simulink model "q_as_mpc"  (R2019a)
settings: Solver=ode1  StartTime=0.0  StopTime=inf  FixedStep=0.001  RelTol=1e-3  EnableMultiTasking=on
values from neighbouring files (symbols this model uses):
  A = [ 0 1 0 -1 ... (first row only)    [setup_as.m]
  B = [0  0 ; 0 1/ms ; -1  0 ; bus/mu -1/mu ]    [setup_as.m]
  C = [ 1 0 0 0 ; -ks/ms -bs/ms 0 bs/ms]    [setup_as.m]
  D = zeros(2,2); D(2,2)=1/ms    [setup_as.m]
  K = lqr( A, B(:,2), Q, R )    [setup_as.m]
  umax = -umin    (= 30)    [setup_as.m]
  umin = -30    [setup_as.m]
  wt_u = R    [setup_as.m]
  wt_y = diag(Q)'    [setup_as.m]
  ymax = -ymin    [setup_as.m]
undefined symbols (not defined in the file or in its folder): HIL, K_d, K_p, qc_get_step_size, ymin
libraries: quarc_library x9, simulink x3, mpclib x2
settings Model: SimulationMode=external  ExtModeTrigDuration=50000  Creator=DCrymble  LastModifiedBy=jxs210080
settings SolverCC: PositivePriorityOrder=on  AutoInsertRateTranBlk=on
settings DataIOCC: LimitDataPoints=on  SaveFormat=Array  SignalLoggingSaveFormat=ModelDataLogs  ReturnWorkspaceOutputs=off
settings OptimizationCC: BooleanDataType=off  OptimizeBlockIOStorage=off  BufferReuse=off  GlobalBufferReuse=off  ExpressionFolding=off  ExpressionDepthLimit=2147483647  LocalBlockOutputs=off  InitFltsAndDblsToZero=on  LifeSpan=inf  OptimizeDataStoreBuffers=off  BusAssignmentInplaceUpdate=off
settings DebuggingCC: UnderspecifiedInitializationDetection=Classic  MergeDetectMultiDrivingBlocksExec=none  SolverPrmCheckMsg=warning  FcnCallInpInsideContextMsg=warning  StateNameClashWarn=warning  SFUnexpectedBacktrackingDiag=warning  SFNoUnconditionalDefaultTransitionDiag=warning  ArithmeticOperatorsInVariantConditions=warning
settings HardwareCC: ProdBitPerPointer=32  ProdBitPerSizeT=32  ProdBitPerPtrDiffT=32  ProdLargestAtomicFloat=None  ProdIntDivRoundTo=Undefined  ProdEndianess=Unspecified  ProdWordSize=32  ProdHWDeviceType=32-bit Generic
settings ModelReferenceCC: PropagateSignalLabelsOutOfModel=off
settings SFSimCC: SimUseLocalCustomCode=off  SimParseCustomCode=off
settings RTWCC: SystemTargetFile=quarc_windows.tlc  TemplateMakefile=quarc_default_tmf  Description=QuaRC Win32 Target  RTWUseLocalCustomCode=off
settings CodeAppCC: StateflowObjectComments=on
settings STFCustomTargetCC: TargetPreCompLibLocation=C:\PROGRA~3\QUARC\lib\2019a\windows\release  ConcurrentExecutionCompliant=on  GeneratePreprocessorConditionals=Disable all  CPPClassGenCompliant=on  SystemTargetFile=quarc_windows.tlc
settings GRTTargetCC: TargetPreCompLibLocation=C:\PROGRA~3\QUARC\lib\2019a\windows\release  TargetLangStandard=C89/C90 (ANSI)  ParMdlRefBuildCompliant=off  CompOptLevelCompliant=off  GeneratePreprocessorConditionals=Disable all  CombineOutputUpdateFcns=off  MatFileLogging=off  GRTInterface=on  UseToolchainInfoCompliant=off  ExtMode=on  ExtModeMexFile=quarc_comm
settings ConfigComp: CovMetricSettings=dw  CovHtmlReporting=on  CovSaveCumulativeToWorkspaceVar=on  CovSaveSingleToWorkspaceVar=on  CovExternalEMLEnable=off

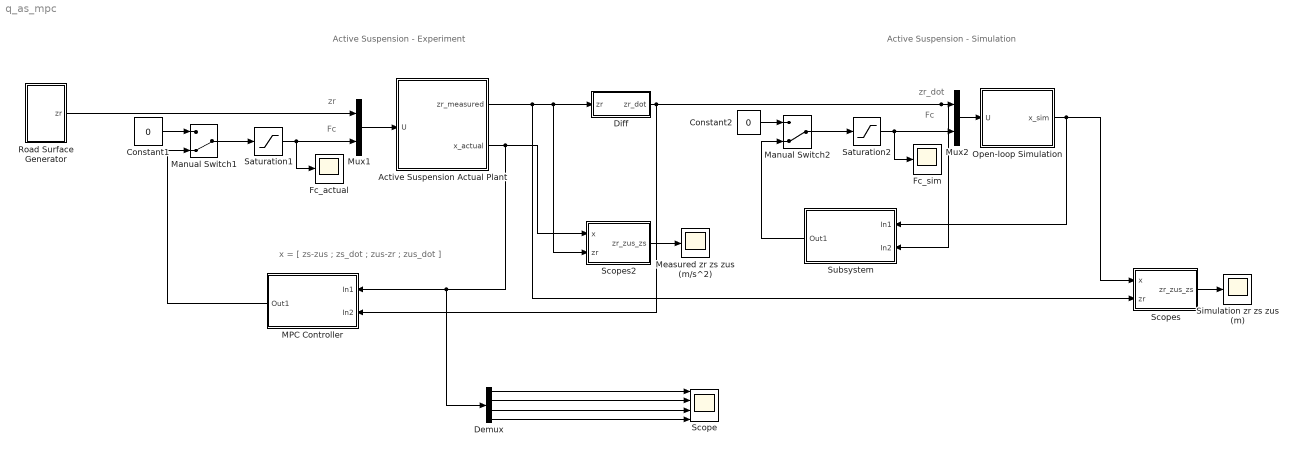
== system q_as_mpc ==
  note: Active Suspension - Experiment
  note: zr
  note: Fc
  note: zr_dot
  note: Fc
  note: x = [ zs-zus ; zs_dot ; zus-zr ; zus_dot ]
  note: Active Suspension - Simulation
  Active Suspension Actual Plant : Subsystem
  Constant1 : Constant  Value=0
  Constant2 : Constant  Value=0
  Demux : Demux
  Diff : Subsystem
  Fc_actual : Scope
  Fc_sim : Scope
  MPC Controller : Subsystem  VariantControl=Variant1
  Manual Switch1 : ManualSwitch  CurrentSetting=0
  Manual Switch2 : ManualSwitch  CurrentSetting=0
  Measured zr zs zus (m/s^2) : Scope
  Mux1 : Mux  Inputs=2
  Mux2 : Mux  Inputs=2
  Open-loop Simulation : Subsystem
  Road Surface Generator : Subsystem
  Saturation1 : Saturate  UpperLimit=38.3  LowerLimit=-38.3
  Saturation2 : Saturate  UpperLimit=39.2  LowerLimit=-39.2
  Scope : Scope  NumInputPorts=4
  Scopes : Subsystem
  Scopes2 : Subsystem
  Simulation zr zs zus (m) : Scope
  Subsystem : Subsystem  VariantControl=Variant1
  wires:
  Road Surface Generator/1(zr) -> Mux1/1
  Manual Switch1/1 -> Saturation1/1
  Mux1/1 -> Active Suspension Actual Plant/1(U)
  Constant1/1 -> Manual Switch1/1
  Saturation1/1 -> Fc_actual/1, Mux1/2
  Constant2/1 -> Manual Switch2/1
  Manual Switch2/1 -> Saturation2/1
  Mux2/1 -> Open-loop Simulation/1(U)
  Scopes2/1(zr_zus_zs) -> Measured zr zs zus (m/s^2)/1
  Scopes/1(zr_zus_zs) -> Simulation zr zs zus (m)/1
  Saturation2/1 -> Mux2/2, Fc_sim/1
  MPC Controller/1(Out1) -> Manual Switch1/2
  Active Suspension Actual Plant/1(zr_measured) -> Scopes/2(zr), Diff/1(zr), Scopes2/2(zr)
  Open-loop Simulation/1(x_sim) -> Subsystem/1(In1), Scopes/1(x)
  Diff/1(zr_dot) -> Subsystem/2(In2), Mux2/1, MPC Controller/2(In2)
  Subsystem/1(Out1) -> Manual Switch2/2
  Active Suspension Actual Plant/2(x_actual) -> Demux/1, MPC Controller/1(In1), Scopes2/1(x)
  Demux/1 -> Scope/1
  Demux/2 -> Scope/2
  Demux/3 -> Scope/3
  Demux/4 -> Scope/4

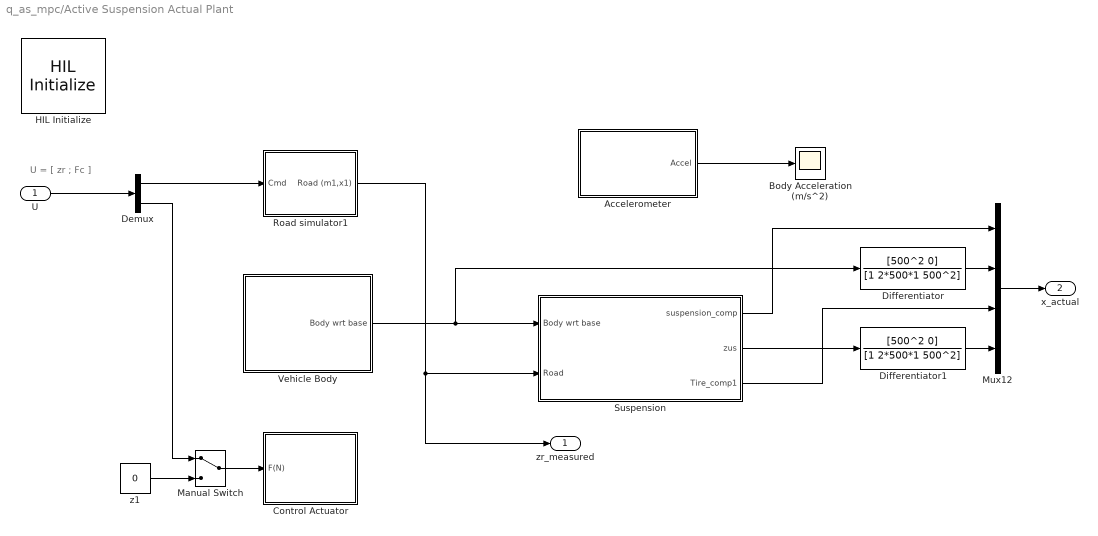
== system q_as_mpc/Active Suspension Actual Plant ==
  note: U = [ zr ; Fc ]
  U : Inport
  Accelerometer : Subsystem
  Body Acceleration (m/s^2) : Scope
  Control Actuator : Subsystem
  Demux : Demux  Outputs=2
  Differentiator : TransferFcn  Numerator=[500^2 0]  Denominator=[1 2*500*1 500^2]
  Differentiator1 : TransferFcn  Numerator=[500^2 0]  Denominator=[1 2*500*1 500^2]
  HIL Initialize : quarc_library/Data Acquisition/Generic/Configuration/HIL Initialize  Priority=-99  object_name=HIL-1  board_type=q8_usb  board_number=0  board_options=update_rate=normal;decimation=1  exclusive=off  active=off  hardware_clocks=[0:2]  clock_modes=[]  initial_clock_frequencies=[]  set_clock_params_at_start=off  set_clock_params_at_switch_in=off  set_clock_frequencies_at_start=off  set_clock_frequencies_at_switch_in=off  analog_input_channels=[0:7]  analog_input_configurations=[]  analog_input_maximums=10  analog_input_minimums=-10  set_analog_input_params_at_start=on  set_analog_input_params_at_switch_in=off  analog_output_channels=[0:7]  analog_output_maximums=10  analog_output_minimums=-10  initial_analog_outputs=[0]  final_analog_outputs=[0]  watchdog_analog_outputs=0  set_analog_output_params_at_start=on  set_analog_output_params_at_switch_in=off  set_analog_outputs_at_start=on  set_analog_outputs_at_switch_in=off  set_analog_outputs_at_terminate=on  set_analog_outputs_at_switch_out=off  set_analog_outputs_on_watchdog=off  digital_input_channels=[]  digital_output_channels=[0:4]  digital_output_configuration=[]  initial_digital_outputs=[0 0 0 0 1]  final_digital_outputs=[1 1 1 1 0]  watchdog_digital_outputs=1  set_digital_output_params_at_start=off  set_digital_output_params_at_switch_in=off  set_digital_outputs_at_start=on  set_digital_outputs_at_switch_in=off  set_digital_outputs_at_terminate=on  set_digital_outputs_at_switch_out=off  set_digital_outputs_on_watchdog=off  encoder_channels=[0:7]  quadrature=[4]  encoder_filter_frequency=[]  initial_encoder_counts=[0]  set_encoder_params_at_start=on  set_encoder_params_at_switch_in=off  set_encoder_counts_at_start=on  set_encoder_counts_at_switch_in=off  pwm_channels=[0:7]  pwm_modes=0  pwm_frequency=99.532799999999995e6/4095  pwm_configuration=[0]  pwm_alignment=[0]  pwm_polarity=[1]  pwm_leading_deadband=[0]  pwm_trailing_deadband=[0]  initial_pwm_outputs=[0]  final_pwm_outputs=[0]  watchdog_pwm_outputs=[0]  set_pwm_params_at_start=on  set_pwm_params_at_switch_in=off  set_pwm_outputs_at_start=on  set_pwm_outputs_at_switch_in=off  set_pwm_outputs_at_terminate=on  set_pwm_outputs_at_switch_out=off  set_pwm_outputs_on_watchdog=off  other_output_channels=[]  initial_other_outputs=[]  final_other_outputs=[]  watchdog_other_outputs=[]  set_other_outputs_at_start=off  set_other_outputs_at_switch_in=off  set_other_outputs_at_terminate=off  set_other_outputs_at_switch_out=off  set_other_outputs_on_watchdog=off
  Manual Switch : ManualSwitch
  Mux12 : Mux
  Road simulator1 : Subsystem
  Suspension : Subsystem
  Vehicle Body : Subsystem
  z1 : Constant  Value=0
  zr_measured : Outport
  x_actual : Outport  Port=2
  wires:
  Manual Switch/1 -> Control Actuator/1(F(N))
  z1/1 -> Manual Switch/2
  Suspension/1(suspension_comp) -> Mux12/1
  Vehicle Body/1(Body wrt base) -> Differentiator/1, Suspension/1("Body wrt base ")
  Differentiator/1 -> Mux12/2
  Differentiator1/1 -> Mux12/4
  Suspension/2(zus) -> Differentiator1/1
  Mux12/1 -> x_actual/1
  Suspension/3(Tire_comp1) -> Mux12/3
  U/1 -> Demux/1
  Road simulator1/1(Road (m1,x1)) -> zr_measured/1, Suspension/2(Road)
  Demux/1 -> Road simulator1/1(Cmd)
  Demux/2 -> Manual Switch/1
  Accelerometer/1(Accel) -> Body Acceleration (m/s^2)/1

== system q_as_mpc/Diff ==
  zr : Inport
  2nd Order Filter Input ICs3 : Subsystem
  Constant3 : Constant  Value=1000
  Terminator_1 : Terminator
  z4 : Constant
  zr_dot : Outport
  wires:
  Constant3/1 -> 2nd Order Filter Input ICs3/2(Wn)
  z4/1 -> 2nd Order Filter Input ICs3/3(z)
  zr/1 -> 2nd Order Filter Input ICs3/1(In)
  2nd Order Filter Input ICs3/2(Out_dot) -> zr_dot/1
  2nd Order Filter Input ICs3/1(Out) -> Terminator_1/1

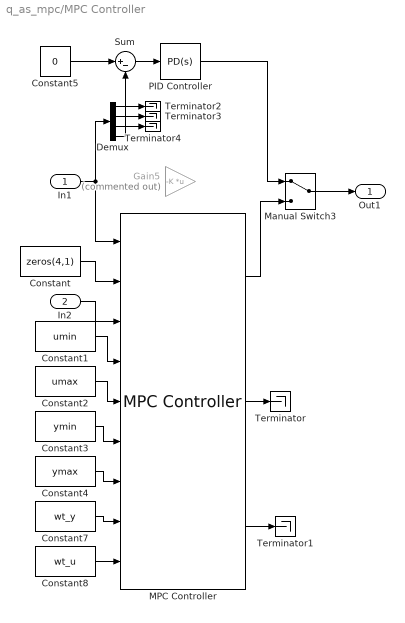
== system q_as_mpc/MPC Controller ==
  In1 : Inport
  In2 : Inport  Port=2
  Constant : Constant  Value=zeros(4,1)
  Constant1 : Constant  Value=umin
  Constant2 : Constant  Value=umax
  Constant3 : Constant  Value=ymin
  Constant4 : Constant  Value=ymax
  Constant5 : Constant  Value=0
  Constant7 : Constant  Value=wt_y
  Constant8 : Constant  Value=wt_u
  Demux : Demux
  Gain5 : Gain  Commented=on  Gain=-K  Multiplication=Matrix(K*u)
  MPC Controller : mpclib/MPC Controller  SCDEnableBlockLinearizationSpecification=on  mpcobj=ctr_mpc  is_multiple=0  enable_value=0  return_u0=off  updateMPCinCallerWorkspace=on  md_inport=on  mv_inport=off  uref_inport=off  return_cost=off  return_mvseq=on  return_qpstatus=off  return_xseq=off  return_state=off  return_ovseq=on  state_inport=off  umin_inport=on  umax_inport=on  ymin_inport=on  ymax_inport=on  cc_inport=off  ywt_inport=on  uwt_inport=on  duwt_inport=off  rhoeps_inport=off  pm_inport=off  MaximumP=100  HorizonChoice=FixedHorizon  n_ts=0.01  n_p=20  n_mv=1  n_md=1  n_ud=0  n_mo=4  n_uo=0  BlockDataType=double  SampleTimeInherited=off  switch_inport=off
      settings: SourceProductName=MATLAB Runtime - Model Predictive Control Toolbox Addin  SourceProductBaseCode=Missing
  Manual Switch3 : ManualSwitch
  PID Controller : simulink/Continuous/PID Controller  Controller=PD  Form=Parallel  TimeDomain=Continuous-time  SampleTime=-1  IntegratorMethod=Forward Euler  FilterMethod=Forward Euler  ControllerParametersSource=internal  P=K_p  I=1  D=K_d  UseFilter=on  N=100  TunerSelectOption=Transfer Function Based (PID Tuner App)  InitialConditionSource=internal  InitialConditionForIntegrator=0  InitialConditionForFilter=0  DifferentiatorICPrevScaledInput=0  ExternalReset=none  TrackingMode=off  Kt=1  LimitOutput=off  UpperSaturationLimit=inf  LowerSaturationLimit=-inf  LinearizeAsGain=on  AntiWindupMode=none  Kb=1  POutMin=[]  POutMax=[]  IOutMin=[]  IOutMax=[]  DOutMin=[]  DOutMax=[]  NOutMin=[]  NOutMax=[]  SumOutMin=[]  SumOutMax=[]  SaturationOutMin=[]  SaturationOutMax=[]  PParamMin=[]  PParamMax=[]  IParamMin=[]  IParamMax=[]  DParamMin=[]  DParamMax=[]  NParamMin=[]  NParamMax=[]  KbParamMin=[]  KbParamMax=[]  KtParamMin=[]  KtParamMax=[]  KbOutMin=[]  KbOutMax=[]  KtOutMin=[]  KtOutMax=[]  IntegratorOutMin=[]  IntegratorOutMax=[]  FilterOutMin=[]  FilterOutMax=[]  SumI1OutMin=[]  SumI1OutMax=[]  SumI2OutMin=[]  SumI2OutMax=[]  SumI3OutMin=[]  SumI3OutMax=[]  SumI4OutMin=[]  SumI4OutMax=[]  SumDOutMin=[]  SumDOutMax=[]  DifferentiatorOutMin=[]  DifferentiatorOutMax=[]  FilterDiffOutCoefMin=[]  FilterDiffOutCoefMax=[]  ReciprocalOutMin=[]  ReciprocalOutMax=[]  SumDenOutMin=[]  SumDenOutMax=[]  SumNumOutMin=[]  SumNumOutMax=[]  DivideOutMin=[]  DivideOutMax=[]  IntegratorContinuousStateAttributes=''  IntegratorStateMustResolveToSignalObject=off  IntegratorRTWStateStorageClass=Auto  FilterContinuousStateAttributes=''  FilterStateMustResolveToSignalObject=off  FilterRTWStateStorageClass=Auto  ParallelPVariant=InternalParameters  IdealPVariant=Disabled  IVariant=Disabled  DVariant=InternalParameters  IntegratorVariant=Disabled  SatVariant=Disabled  AWVariant=Disabled  PCopyVariant=Disabled  TRVariant=Disabled  FdbkBlocksVariant=Forward  IdealPFdbkVariant=Disabled  SatFdbkVariant=Disabled  DerivativeFilterVariant=ContFilter  NVariant=InternalParameters  NCopyVariant=Disabled  FilterICVariant=InternalICsFilter  IntegratorICVariant=Disabled  ExternalResetVariant=Disabled  TRSumVariant=Passthrough  SumFdbkVariant=Disabled  SumVariant=Sum_PD
  Sum : Sum  Inputs=|+-
  Terminator{,1..4} (5 alike) : Terminator
  Out1 : Outport
  wires:
  In2/1 -> MPC Controller/3
  Constant1/1 -> MPC Controller/4
  Manual Switch3/1 -> Out1/1
  Constant8/1 -> MPC Controller/9
  Constant7/1 -> MPC Controller/8
  Constant4/1 -> MPC Controller/7
  Constant3/1 -> MPC Controller/6
  Constant2/1 -> MPC Controller/5
  In1/1 -> Demux/1, MPC Controller/1
  Constant/1 -> MPC Controller/2
  MPC Controller/1 -> Manual Switch3/2
  MPC Controller/2 -> Terminator/1
  MPC Controller/3 -> Terminator1/1
  Constant5/1 -> Sum/1
  Sum/1 -> PID Controller/1
  Demux/4 -> Sum/2
  PID Controller/1 -> Manual Switch3/1
  Demux/1 -> Terminator2/1
  Demux/2 -> Terminator3/1
  Demux/3 -> Terminator4/1

== system q_as_mpc/Open-loop Simulation ==
  U : Inport
  Demux : Demux  Outputs=[4 2]
  Open-Loop State-Space : StateSpace  A=A  B=B  C=cat(1,eye(4), C)  D=cat(1,zeros(4,2),D)  InitialCondition=0
  Terminator : Terminator
  Unit Delay : UnitDelay  SampleTime=-1  HasFrameUpgradeWarning=on
  x_sim : Outport
  wires:
  Open-Loop State-Space/1 -> Demux/1
  Demux/1 -> Unit Delay/1
  U/1 -> Open-Loop State-Space/1
  Unit Delay/1 -> x_sim/1
  Demux/2 -> Terminator/1

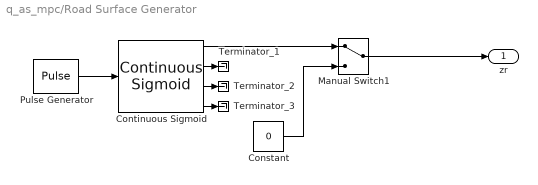
== system q_as_mpc/Road Surface Generator ==
  Constant : Constant  Value=0
  Continuous Sigmoid : quarc_library/Sources/Sigmoids/Continuous Sigmoid  params_source=Internal (dialog parameters)  max_velocity=.6/3  max_acceleration=20  initial_position=0  initial_velocity=0  hold_off=0.5  input_sample_time=-1  output_sample_time=qc_get_step_size
      settings: SourceProductName=QUARC Targets
  Manual Switch1 : ManualSwitch
  Pulse Generator : DiscretePulseGenerator  PulseType=Time based  Amplitude=0.02  Period=3  PulseWidth=50  PhaseDelay=.1
  Terminator_1 : Terminator
  Terminator_2 : Terminator
  Terminator_3 : Terminator
  zr : Outport
  wires:
  Pulse Generator/1 -> Continuous Sigmoid/1
  Constant/1 -> Manual Switch1/2
  Continuous Sigmoid/2 -> Terminator_1/1
  Continuous Sigmoid/3 -> Terminator_2/1
  Continuous Sigmoid/4 -> Terminator_3/1
  Manual Switch1/1 -> zr/1
  Continuous Sigmoid/1 -> Manual Switch1/1

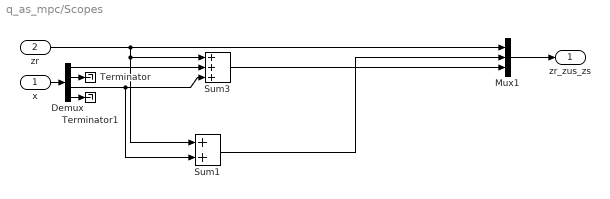
== system q_as_mpc/Scopes ==
  x : Inport
  zr : Inport  Port=2
  Demux : Demux
  Mux1 : Mux  Inputs=3
  Sum1 : Sum  Inputs=2  SaturateOnIntegerOverflow=on  InputSameDT=on  OutDataTypeStr=Inherit: Same as first input
  Sum3 : Sum  Inputs=3  SaturateOnIntegerOverflow=on  InputSameDT=on  OutDataTypeStr=Inherit: Same as first input
  Terminator : Terminator
  Terminator1 : Terminator
  zr_zus_zs : Outport
  wires:
  Demux/1 -> Sum3/2
  Demux/3 -> Sum3/3, Sum1/2
  zr/1 -> Mux1/1, Sum3/1, Sum1/1
  x/1 -> Demux/1
  Sum1/1 -> Mux1/2
  Sum3/1 -> Mux1/3
  Mux1/1 -> zr_zus_zs/1
  Demux/2 -> Terminator/1
  Demux/4 -> Terminator1/1

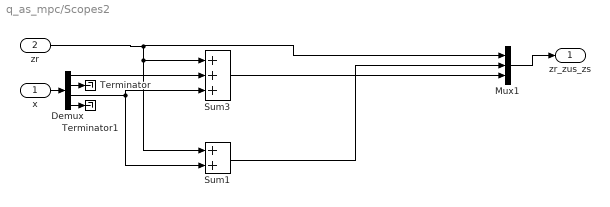
== system q_as_mpc/Scopes2 ==
  x : Inport
  zr : Inport  Port=2
  Demux : Demux
  Mux1 : Mux  Inputs=3
  Sum1 : Sum  Inputs=2  SaturateOnIntegerOverflow=on  InputSameDT=on  OutDataTypeStr=Inherit: Same as first input
  Sum3 : Sum  Inputs=3  SaturateOnIntegerOverflow=on  InputSameDT=on  OutDataTypeStr=Inherit: Same as first input
  Terminator : Terminator
  Terminator1 : Terminator
  zr_zus_zs : Outport
  wires:
  Mux1/1 -> zr_zus_zs/1
  Sum3/1 -> Mux1/3
  Sum1/1 -> Mux1/2
  x/1 -> Demux/1
  zr/1 -> Sum1/1, Sum3/1, Mux1/1
  Demux/3 -> Sum1/2, Sum3/3
  Demux/1 -> Sum3/2
  Demux/2 -> Terminator/1
  Demux/4 -> Terminator1/1

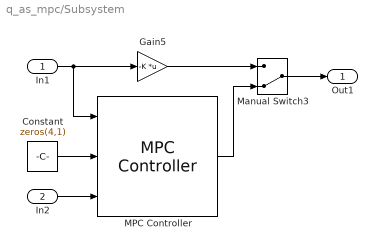
== system q_as_mpc/Subsystem ==
  In1 : Inport
  In2 : Inport  Port=2
  Constant : Constant  Value=zeros(4,1)
  Gain5 : Gain  Gain=-K  Multiplication=Matrix(K*u)
  MPC Controller : mpclib/MPC Controller  SCDEnableBlockLinearizationSpecification=on  mpcobj=ctr_mpc  is_multiple=0  enable_value=0  return_u0=off  updateMPCinCallerWorkspace=on  md_inport=on  mv_inport=off  uref_inport=off  return_cost=off  return_mvseq=off  return_qpstatus=off  return_xseq=off  return_state=off  return_ovseq=off  state_inport=off  umin_inport=off  umax_inport=off  ymin_inport=off  ymax_inport=off  cc_inport=off  ywt_inport=off  uwt_inport=off  duwt_inport=off  rhoeps_inport=off  pm_inport=off  MaximumP=10  HorizonChoice=FixedHorizon  n_ts=0.01  n_p=20  n_mv=1  n_md=1  n_ud=0  n_mo=4  n_uo=0  BlockDataType=double  SampleTimeInherited=off  switch_inport=off
      settings: SourceProductName=MATLAB Runtime - Model Predictive Control Toolbox Addin  SourceProductBaseCode=Missing
  Manual Switch3 : ManualSwitch  CurrentSetting=0
  Out1 : Outport
  wires:
  In2/1 -> MPC Controller/3
  Constant/1 -> MPC Controller/2
  MPC Controller/1 -> Manual Switch3/2
  Gain5/1 -> Manual Switch3/1
  In1/1 -> Gain5/1, MPC Controller/1
  Manual Switch3/1 -> Out1/1

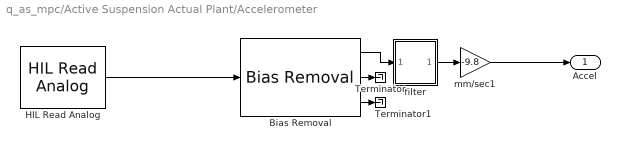
== system q_as_mpc/Active Suspension Actual Plant/Accelerometer ==
  Bias Removal : quarc_library/Discrete/Bias Removal  start_time=0  end_time=.099  switch_id=0  sample_time=qc_get_step_size
      settings: SourceProductName=QUARC Targets
  HIL Read Analog : quarc_library/Data Acquisition/Generic/Immediate I//O/HIL Read Analog  object_name=HIL-1  channels=0  sample_time=qc_get_step_size  active=on  vector_output=off
  Terminator : Terminator
  Terminator1 : Terminator
  filter : Subsystem
  mm/sec1 : Gain  Gain=-9.8
  Accel : Outport
  wires:
  Bias Removal/1 -> filter/1(In1)
  filter/1(Out2) -> mm/sec1/1
  mm/sec1/1 -> Accel/1
  HIL Read Analog/1 -> Bias Removal/1
  Bias Removal/2 -> Terminator/1
  Bias Removal/3 -> Terminator1/1

== system q_as_mpc/Active Suspension Actual Plant/Control Actuator ==
  F(N) : Inport
  A/V : Gain  Gain=-2
  A/V1 : Gain  Gain=1/19.16
  Amp : Scope
  Force : Scope
  HIL Write Analog1 : quarc_library/Data Acquisition/Generic/Immediate I//O/HIL Write Analog  object_name=HIL-1  channels=0  sample_time=-1  active=off  vector_input=on
  Saturation2 : Saturate  UpperLimit=5  LowerLimit=-5
  wires:
  Saturation2/1 -> Amp/1, A/V/1
  A/V1/1 -> Saturation2/1
  F(N)/1 -> Force/1, A/V1/1
  A/V/1 -> HIL Write Analog1/1

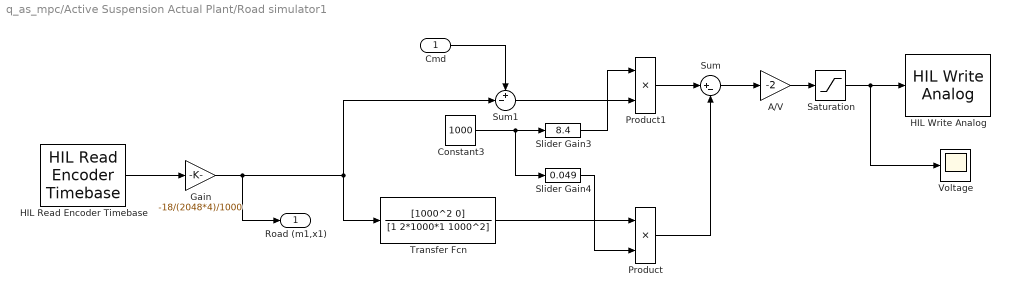
== system q_as_mpc/Active Suspension Actual Plant/Road simulator1 ==
  Cmd : Inport
  A/V : Gain  Gain=-2
  Constant3 : Constant  Value=1000
  Gain : Gain  Gain=-18/(2048*4)/1000
  HIL Read Encoder Timebase : quarc_library/Data Acquisition/Generic/Timebases/HIL Read Encoder Timebase  object_name=HIL-1  clock=[0]  channels=1  samples_in_buffer=max(ceil(1/qc_get_step_size), 1)  active=on  vector_output=on  data_type_mode=Inherit via back propagation  data_type=double
  HIL Write Analog : quarc_library/Data Acquisition/Generic/Immediate I//O/HIL Write Analog  object_name=HIL-1  channels=1  sample_time=-1  active=off  vector_input=on
  Product : Product  RndMeth=Zero
  Product1 : Product  RndMeth=Zero
  Saturation : Saturate  UpperLimit=10  LowerLimit=-10
  Slider Gain3 : simulink/Math Operations/Slider Gain  gain=8.4  low=0  high=70
  Slider Gain4 : simulink/Math Operations/Slider Gain  gain=0.049  low=0  high=0.1
  Sum : Sum  Inputs=|+-
  Sum1 : Sum  Inputs=+-|
  Transfer Fcn : TransferFcn  Numerator=[1000^2 0]  Denominator=[1 2*1000*1 1000^2]
  Voltage : Scope
  Road (m1,x1) : Outport
  wires:
  A/V/1 -> Saturation/1
  Constant3/1 -> Slider Gain4/1, Slider Gain3/1
  HIL Read Encoder Timebase/1 -> Gain/1
  Saturation/1 -> HIL Write Analog/1, Voltage/1
  Sum/1 -> A/V/1
  Gain/1 -> Road (m1,x1)/1, Transfer Fcn/1, Sum1/2
  Transfer Fcn/1 -> Product/1
  Slider Gain3/1 -> Product1/1
  Sum1/1 -> Product1/2
  Product1/1 -> Sum/1
  Slider Gain4/1 -> Product/2
  Product/1 -> Sum/2
  Cmd/1 -> Sum1/1

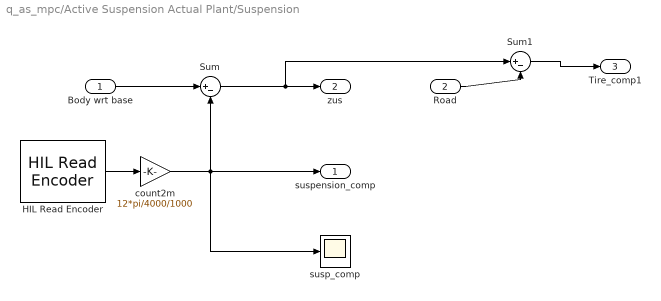
== system q_as_mpc/Active Suspension Actual Plant/Suspension ==
  "Body wrt base " : Inport
  Road : Inport  Port=2
  HIL Read Encoder : quarc_library/Data Acquisition/Generic/Immediate I//O/HIL Read Encoder  object_name=HIL-1  channels=0  sample_time=qc_get_step_size  active=on  vector_output=off  data_type_mode=Inherit via back propagation  data_type=double
  Sum : Sum  Inputs=|+-
  Sum1 : Sum  Inputs=|+-
  count2m : Gain  Gain=12*pi/4000/1000
  susp_comp : Scope
  suspension_comp : Outport
  zus : Outport  Port=2
  Tire_comp1 : Outport  Port=3
  wires:
  Sum/1 -> zus/1, Sum1/1
  "Body wrt base "/1 -> Sum/1
  HIL Read Encoder/1 -> count2m/1
  count2m/1 -> Sum/2, suspension_comp/1, susp_comp/1
  Road/1 -> Sum1/2
  Sum1/1 -> Tire_comp1/1

== system q_as_mpc/Active Suspension Actual Plant/Vehicle Body ==
  Body wrt base1 : Scope
  HIL Read Encoder : quarc_library/Data Acquisition/Generic/Immediate I//O/HIL Read Encoder  object_name=HIL-1  channels=2  sample_time=qc_get_step_size  active=on  vector_output=off  data_type_mode=Inherit via back propagation  data_type=double
  count2m : Gain  Gain=pi()*25.4/4/4096/1000
  Body wrt base : Outport
  wires:
  HIL Read Encoder/1 -> count2m/1
  count2m/1 -> Body wrt base/1, Body wrt base1/1

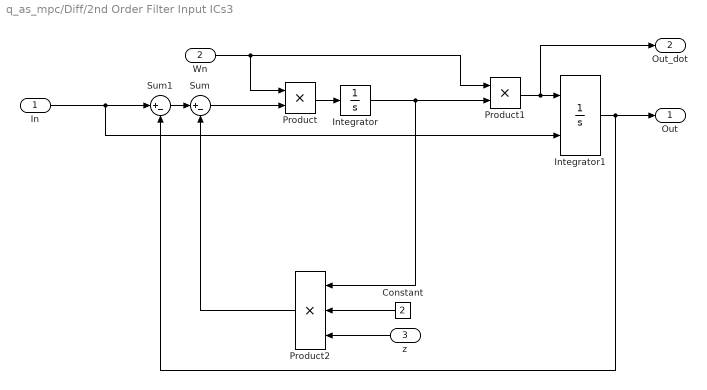
== system q_as_mpc/Diff/2nd Order Filter Input ICs3 ==
  In : Inport
  Wn : Inport  Port=2
  z : Inport  Port=3
  Constant : Constant  Value=2
  Integrator : Integrator
  Integrator1 : Integrator  InitialConditionSource=external
  Product : Product  RndMeth=Zero
  Product1 : Product  RndMeth=Zero
  Product2 : Product  Inputs=3  RndMeth=Zero
  Sum : Sum  Inputs=|+-
  Sum1 : Sum  Inputs=|+-
  Out : Outport
  Out_dot : Outport  Port=2
  wires:
  Constant/1 -> Product2/2
  z/1 -> Product2/3
  Product2/1 -> Sum/2
  In/1 -> Integrator1/2, Sum1/1
  Sum1/1 -> Sum/1
  Integrator1/1 -> Out/1, Sum1/2
  Integrator/1 -> Product2/1, Product1/2
  Product1/1 -> Out_dot/1, Integrator1/1
  Wn/1 -> Product1/1, Product/1
  Sum/1 -> Product/2
  Product/1 -> Integrator/1

== system q_as_mpc/Active Suspension Actual Plant/Accelerometer/filter ==
  In1 : Inport
  2nd Order Filter Input ICs3 : Subsystem
  Constant3 : Constant  Value=70
  Terminator_1 : Terminator
  z4 : Constant
  Out2 : Outport
  wires:
  In1/1 -> 2nd Order Filter Input ICs3/1(In)
  z4/1 -> 2nd Order Filter Input ICs3/3(z)
  Constant3/1 -> 2nd Order Filter Input ICs3/2(Wn)
  2nd Order Filter Input ICs3/1(Out) -> Out2/1
  2nd Order Filter Input ICs3/2(Out_dot) -> Terminator_1/1

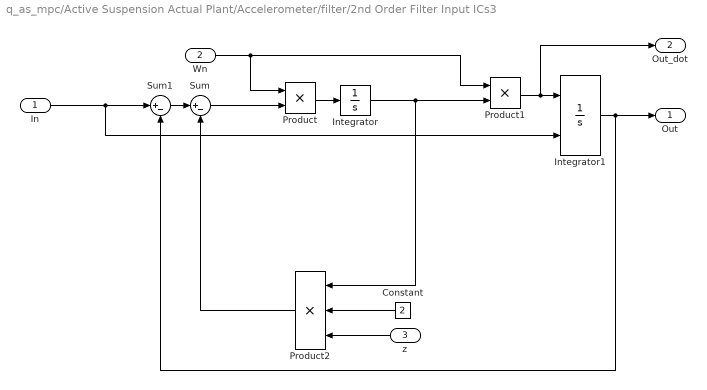
== system q_as_mpc/Active Suspension Actual Plant/Accelerometer/filter/2nd Order Filter Input ICs3 ==
  In : Inport
  Wn : Inport  Port=2
  z : Inport  Port=3
  Constant : Constant  Value=2
  Integrator : Integrator
  Integrator1 : Integrator  InitialConditionSource=external
  Product : Product  RndMeth=Zero
  Product1 : Product  RndMeth=Zero
  Product2 : Product  Inputs=3  RndMeth=Zero
  Sum : Sum  Inputs=|+-
  Sum1 : Sum  Inputs=|+-
  Out : Outport
  Out_dot : Outport  Port=2
  wires:
  Constant/1 -> Product2/2
  z/1 -> Product2/3
  Product2/1 -> Sum/2
  In/1 -> Integrator1/2, Sum1/1
  Sum1/1 -> Sum/1
  Integrator1/1 -> Out/1, Sum1/2
  Integrator/1 -> Product2/1, Product1/2
  Product1/1 -> Out_dot/1, Integrator1/1
  Wn/1 -> Product1/1, Product/1
  Sum/1 -> Product/2
  Product/1 -> Integrator/1
